simulink model "simulacion"  (R2021a)
settings: Solver=VariableStepAuto  StartTime=0.0  StopTime=20  RelTol=1e-3
values from neighbouring files (symbols this model uses):
  Gs = n*KI*180/pi/Jeq/(s+KI^2/Jeq)    [desarrollo.m]
  Jeq = Jm+n^2*JL    [desarrollo.m]
  K = -polyval(Gs.den{1},polo_des)/polyval(Gs.num{1},polo_des)    [desarrollo.m]
  Kd = -polyval(Gla.den{1},polo_des)/polyval(Gla.num{1},polo_des)    [desarrollo.m]
  KI = den(end)/num(end)    [desarrollo.m]
  Kp = Kd*zero    [desarrollo.m]
  Ts_theta = 0.2061    [desarrollo.m]
  Ts_w = 0.0391    [desarrollo.m]
settings Model: Creator=pierr  LastModifiedBy=pierr

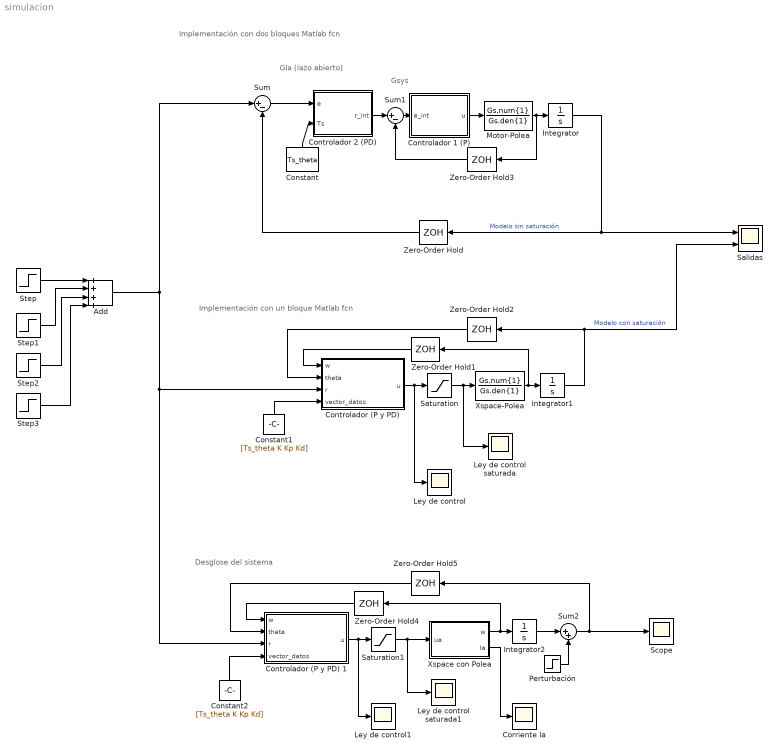
== system simulacion ==
  note: Implementación con dos bloques Matlab fcn
  note: Gla (lazo abierto)
  note: Gsys
  note: Implementación con un bloque Matlab fcn
  note: Desglose del sistema
  Add : Sum  Inputs=++++
  Constant : Constant  Value=Ts_theta
  Constant1 : Constant  Value=[Ts_theta K Kp Kd]
  Constant2 : Constant  Value=[Ts_theta K Kp Kd]
  "Controlador (P y PD) " : MATLAB Function  TreatAsAtomicUnit=on
  Controlador (P y PD) 1 : MATLAB Function  TreatAsAtomicUnit=on
  Controlador 1 (P) : MATLAB Function  TreatAsAtomicUnit=on
  Controlador 2 (PD) : MATLAB Function  TreatAsAtomicUnit=on
  Corriente Ia : Scope
  Integrator : Integrator
  Integrator1 : Integrator
  Integrator2 : Integrator
  Ley de control : Scope
  Ley de control saturada : Scope
  Ley de control saturada1 : Scope
  Ley de control1 : Scope
  Motor-Polea : TransferFcn  Numerator=Gs.num{1}  Denominator=Gs.den{1}
  Perturbación : Step  Time=3  After=18  SampleTime=0
  Salidas : Scope  NumInputPorts=2
  Saturation : Saturate  UpperLimit=5  LowerLimit=-5
  Saturation1 : Saturate  UpperLimit=5  LowerLimit=-5
  Scope : Scope
  Step : Step  Time=0  After=180  SampleTime=0
  Step1 : Step  Time=5  After=180  SampleTime=0
  Step2 : Step  Time=10  After=180  SampleTime=0
  Step3 : Step  Time=15  After=180  SampleTime=0
  Sum : Sum  Inputs=|+-
  Sum1 : Sum  Inputs=|+-
  Sum2 : Sum  Inputs=|++
  Xspace con Polea : Subsystem
  Xspace-Polea : TransferFcn  Numerator=Gs.num{1}  Denominator=Gs.den{1}
  Zero-Order Hold : ZeroOrderHold  SampleTime=Ts_theta
  Zero-Order Hold1 : ZeroOrderHold  SampleTime=Ts_w
  Zero-Order Hold2 : ZeroOrderHold  SampleTime=Ts_theta
  Zero-Order Hold3 : ZeroOrderHold  SampleTime=Ts_w
  Zero-Order Hold4 : ZeroOrderHold  SampleTime=Ts_w
  Zero-Order Hold5 : ZeroOrderHold  SampleTime=Ts_theta
  wires:
  Motor-Polea/1 -> Zero-Order Hold3/1, Integrator/1
  Constant/1 -> Controlador 2 (PD)/2(Ts)
  Controlador 1 (P)/1(u) -> Motor-Polea/1
  Controlador 2 (PD)/1(r_int) -> Sum1/1
  Sum1/1 -> Controlador 1 (P)/1(e_int)
  Sum/1 -> Controlador 2 (PD)/1(e)
  Integrator/1 -> Zero-Order Hold/1, Salidas/1  "Modelo sin saturación"
  Zero-Order Hold/1 -> Sum/2
  Xspace-Polea/1 -> Zero-Order Hold1/1, Integrator1/1
  Integrator1/1 -> Zero-Order Hold2/1, Salidas/2  "Modelo con saturación"
  Constant1/1 -> "Controlador (P y PD) "/4(vector_datos)
  Zero-Order Hold1/1 -> "Controlador (P y PD) "/1(w)
  Zero-Order Hold2/1 -> "Controlador (P y PD) "/2(theta)
  Zero-Order Hold3/1 -> Sum1/2
  Saturation/1 -> Ley de control saturada/1, Xspace-Polea/1
  "Controlador (P y PD) "/1(u) -> Saturation/1, Ley de control/1
  Controlador (P y PD) 1/1(u) -> Saturation1/1, Ley de control1/1
  Saturation1/1 -> Xspace con Polea/1(ua), Ley de control saturada1/1
  Xspace con Polea/1(w) -> Integrator2/1, Zero-Order Hold4/1
  Zero-Order Hold4/1 -> Controlador (P y PD) 1/1(w)
  Integrator2/1 -> Sum2/1
  Zero-Order Hold5/1 -> Controlador (P y PD) 1/2(theta)
  Constant2/1 -> Controlador (P y PD) 1/4(vector_datos)
  Add/1 -> Controlador (P y PD) 1/3(r), "Controlador (P y PD) "/3(r), Sum/1
  Xspace con Polea/2(Ia) -> Corriente Ia/1
  Step1/1 -> Add/2
  Step/1 -> Add/1
  Step2/1 -> Add/3
  Step3/1 -> Add/4
  Sum2/1 -> Zero-Order Hold5/1, Scope/1
  Perturbación/1 -> Sum2/2

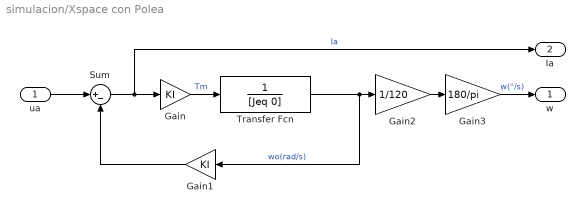
== system simulacion/Xspace con Polea ==
  ua : Inport
  Gain : Gain  Gain=KI
  Gain1 : Gain  Gain=KI
  Gain2 : Gain  Gain=1/120
  Gain3 : Gain  Gain=180/pi
  Sum : Sum  Inputs=|+-
  Transfer Fcn : TransferFcn  Denominator=[Jeq 0]
  w : Outport
  Ia : Outport  Port=2
  wires:
  Sum/1 -> Gain/1, Ia/1  "Ia"
  Gain1/1 -> Sum/2
  Gain/1 -> Transfer Fcn/1  "Tm"
  ua/1 -> Sum/1
  Transfer Fcn/1 -> Gain1/1, Gain2/1  "wo(rad/s)"
  Gain2/1 -> Gain3/1
  Gain3/1 -> w/1  "w(°/s)"

== matlab function simulacion/Controlador 2 (PD) ==
  data: e input; r_int output; Ts input
function r_int = fcn(e,Ts)
persistent e_1
if isempty(e_1)
    e_1=0;
end
Kp=1.329074720803806;
Kd=0.332268680200952;
r_int=Kd/Ts*(e-e_1)+Kp*e;
e_1=e;

== matlab function simulacion/Controlador 1 (P) ==
  data: e_int input; u output
function u = fcn(e_int)
K=0.083308386906803;
u=e_int*K;

== matlab function simulacion/Controlador (P y PD)  ==
  data: w input; theta input; r input; vector_datos input; u output
function u = fcn(w, theta,r,vector_datos)
persistent e1_1
if isempty(e1_1)
    e1_1=0;
end
Ts=vector_datos(1);
K=vector_datos(2);
Kp=vector_datos(3);
Kd=vector_datos(4);
e=r-theta;
r_int=Kd/Ts*(e-e1_1)+Kp*e;
e1_1=e;
e_int=r_int-w;
u=e_int*K;

== matlab function simulacion/Controlador (P y PD) 1 ==
  data: w input; theta input; r input; vector_datos input; u output
function u = fcn(w, theta,r,vector_datos)
persistent e1_1
if isempty(e1_1)
    e1_1=0;
end
Ts=vector_datos(1);
K=vector_datos(2);
Kp=vector_datos(3);
Kd=vector_datos(4);
e=r-theta;
r_int=Kd/Ts*(e-e1_1)+Kp*e;
e1_1=e;
e_int=r_int-w;
u=e_int*K;
